simulink model "receive_a429_r2020b"  (R2020b)
settings: Solver=VariableStepAuto  StartTime=0.0  StopTime=10.0  RelTol=1e-3
libraries: lib_ed247 x2
settings Model: EnablePacing=on  Creator=odufour  LastModifiedBy=odufour

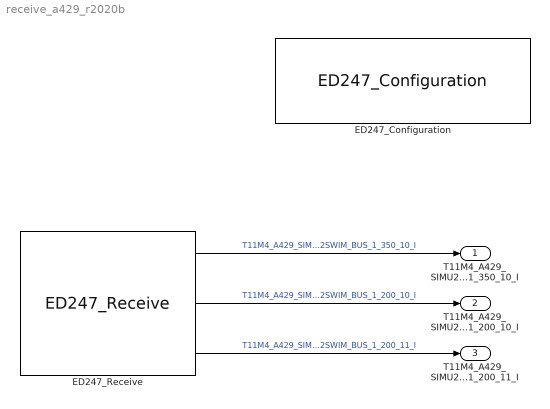
== system receive_a429_r2020b ==
  ED247_Configuration : lib_ed247/ED247_Configuration  configurationFilename='ecic_func_exchange_a429_uc_tester_simple.xml'  enableLog=on  logFilename='<PROJECT_FOLDER>\tests\_files\tmp.log'
      settings: SourceProductName=Airbus ED247
  ED247_Receive : lib_ed247/ED247_Receive  Parameter1=0
      settings: SourceProductName=Airbus ED247
  T11M4_A429_SIMU2SWIM_BUS_1_350_10_I : Outport  OutDataTypeStr=uint8  PortDimensions=4  SampleTime=0.1
  T11M4_A429_SIMU2SWIM_BUS_1_200_10_I : Outport  Port=2  OutDataTypeStr=uint8  PortDimensions=4  SampleTime=0.1
  T11M4_A429_SIMU2SWIM_BUS_1_200_11_I : Outport  Port=3  OutDataTypeStr=uint8  PortDimensions=4  SampleTime=0.1
  wires:
  ED247_Receive/1 -> T11M4_A429_SIMU2SWIM_BUS_1_350_10_I/1  "T11M4_A429_SIMU2SWIM_BUS_1_350_10_I"
  ED247_Receive/2 -> T11M4_A429_SIMU2SWIM_BUS_1_200_10_I/1  "T11M4_A429_SIMU2SWIM_BUS_1_200_10_I"
  ED247_Receive/3 -> T11M4_A429_SIMU2SWIM_BUS_1_200_11_I/1  "T11M4_A429_SIMU2SWIM_BUS_1_200_11_I"
